simulink model "aerosim_simulink_cosim_demo"  (R2024a)
settings: Solver=FixedStepAuto  StartTime=0.0  StopTime=inf  FixedStep=dt_sec  RelTol=1e-3
values from neighbouring files (symbols this model uses):
  altitude_tgt = 0.0    (= 0)    [load_aerosim_simulink_cosim_demo.m]
  dt_sec = 0.02    [load_aerosim_simulink_cosim_demo.m]
libraries: aerosim_simulink_block_library x6, slpidlib x1
settings Model: Creator=ed  LastModifiedBy=Leo.Wong

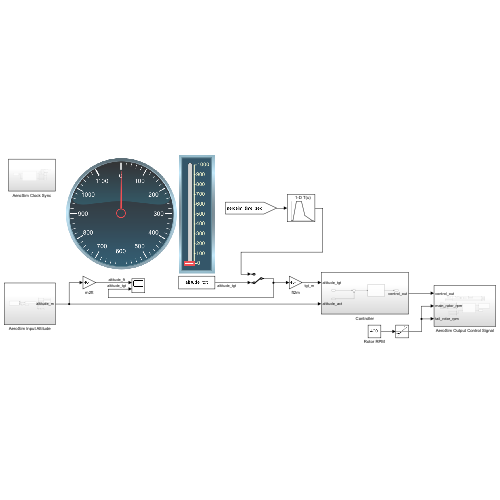
[thumbnail: Simulink's stored preview of the top-level diagram]
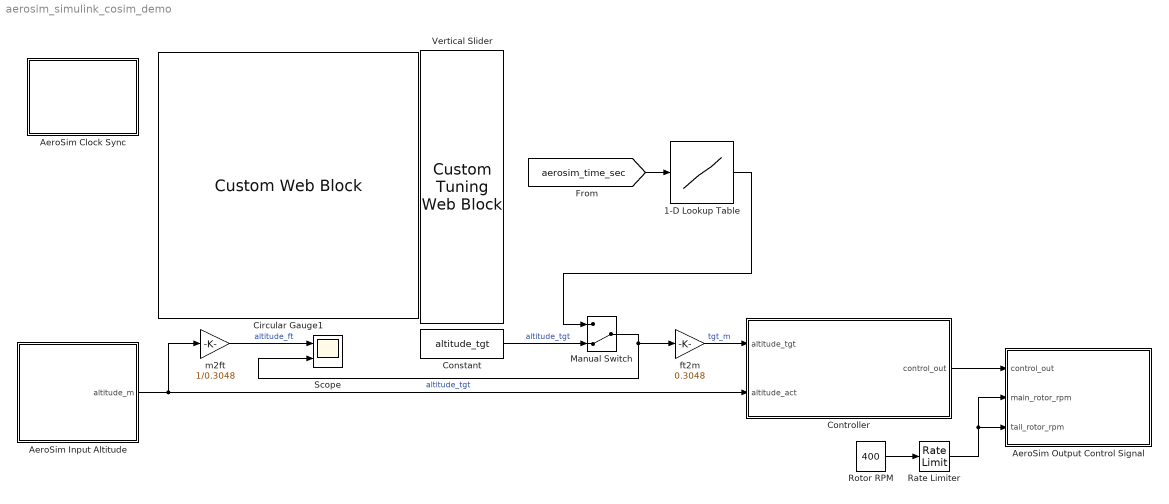
== system aerosim_simulink_cosim_demo ==
  1-D Lookup Table : Lookup_n-D  NumberOfTableDimensions=1  BreakpointsForDimension1=[0;5;15;30;40;60;65]  Table=[0;0;800;800;200;0;0]  ExtrapMethod=Clip  UseLastTableValue=on  InternalRulePriority=Speed  RndMeth=Simplest
  AeroSim Clock Sync : Subsystem  Priority=0
  AeroSim Input Altitude : Subsystem
  AeroSim Output Control Signal : Subsystem
  Circular Gauge1 : CustomWebBlock  LabelPosition=Hide  ShowInitialText=on  Configuration="{\"components\":[{\"name\":\"CircularScaleComponent\",\"settings\":{\"bounds\":{\"max\":1100,\"min\":0,\"tickInterval\":100},\"direction\":\"cw\",\"flipLimits\":0,\"innerRadius\":0.86,\"internalTickHeightScaleFactor\":1,\"labelColor\":[255,255,255],\"labelFont\":{\"font\":\"Arial\",\"fontSize\":12},\"labelRadius\":0.74,\"labelTransparency\":1,\"minorTickHeightScaleFactor\":0.2,\"needleImage\":{\"size\":[200,50],\"src\":\"data:image\\/svg+xml;base64,PD94bWwgdmVyc2lvbj0iMS4wIiBlbmNvZGluZz0idXRmLTgiPz4KPCEtLSBHZW5lcmF0b3I6IEFkb2JlIElsbHVzdHJhdG9yIDI0LjEuMiwgU1ZHIEV4cG9ydCBQbHVnLUluIC4gU1ZHIFZlcnNpb246IDYuMDAgQnVpbGQgMCkgIC0tPgo8c3ZnIHZlcnNpb249IjEuMSIgaWQ9IkxheWVyXzEiIHhtbG5zPSJodHRwOi8vd3d3LnczLm9yZy8yMDAwL3N2ZyIgeG1sbnM6eGxpbms9Imh0dHA6Ly93d3cudzMub3JnLzE5OTkveGxpbmsiIHg9IjBweCIgeT0iMHB4IgoJIHZpZXdCb3g9IjAgMCAyMDAgNTAiIHN0eWxlPSJlbmFibGUtYmFja2dyb3VuZDpuZXcgMCAwIDIwMCA1MDsiIHhtbDpzcGFjZT0icHJlc2VydmUiPgo8c3R5bGUgdHlwZT0idGV4dC9jc3MiPgoJLnN0MHtmaWxsOiNFQzIxMjc7fQo8L3N0eWxlPgo8cGF0aCBjbGFzcz0ic3QwIiBkPSJNMTYyLjgsMTMuN0MxNjksNC40LDE4MS43LDEuOSwxOTEsOC4xczExLjgsMTguOSw1LjYsMjguMnMtMTguOSwxMS44LTI4LjIsNS42bDAsMAoJQzE1OS4xLDM1LjYsMTU2LjYsMjMsMTYyLjgsMTMuN0wxNjIuOCwxMy43eiBNMTY1LjgsMTUuOGMtNS4xLDcuNi0zLjEsMTcuOSw0LjYsMjNjNy42LDUuMSwxNy45LDMuMSwyMy00LjYKCWM1LjEtNy42LDMuMS0xNy45LTQuNi0yM2wwLDBDMTgxLjIsNi4yLDE3MC45LDguMiwxNjUuOCwxNS44eiIvPgo8cGF0aCBjbGFzcz0ic3QwIiBkPSJNMC40LDI1Ljl2LTMuM2wxNTktMi41Yy0wLjcsMi42LTAuNyw1LjIsMCw3LjhMMC40LDI1Ljl6Ii8+CjxjaXJjbGUgY2xhc3M9InN0MCIgY3g9IjE3OS42IiBjeT0iMjQiIHI9IjAuNyIvPgo8L3N2Zz4K\"},\"needleOffset\":[0.18464878250906522,0],\"needleOrientation\":-45,\"needleRotation\":180,\"needleSize\":{\"height\":0.11741692305346914,\"width\":0.46108337545091255},\"outerRadius\":1,\"position\":[0.05,0.05,0.9,0.9],\"referencePoint\":\"auto\",\"scaleAngle\":330,\"scaleAngleOffset\":270,\"scaleColors\":[],\"scaleColorsSize\":0.2,\"scaleDirection\":\"CW\",\"scalePosition\":[0,0,1,1],\"showLabels\":1,\"showMinorTicks\":1,\"showSpanLine\":false,\"showTicks\":true,\"tickColor\":[255,255,255],\"tickTransparency\":1,\"valueBarColor\":[255,255,255],\"valueBarPosition\":[0,0,1,1],\"valueBarSize\":0.2,\"valueBarTransparency\":0.2}},{\"name\":\"BackgroundImageComponent\",\"settings\":{\"image\":{\"size\":[500,500],\"src\":\"data:image\\/svg+xml;base64,PD94bWwgdmVyc2lvbj0iMS4wIiBlbmNvZGluZz0iVVRGLTgiIHN0YW5kYWxvbmU9Im5vIj8+CjxzdmcKICAgeG1sbnM6ZGM9Imh0dHA6Ly9wdXJsLm9yZy9kYy9lbGVtZW50cy8xLjEvIgogICB4bWxuczpjYz0iaHR0cDovL2NyZWF0aXZlY29tbW9ucy5vcmcvbnMjIgogICB4bWxuczpyZGY9Imh0dHA6Ly93d3cudzMub3JnLzE5OTkvMDIvMjItcmRmLXN5bnRheC1ucyMiCiAgIHhtbG5zOnN2Zz0iaHR0cDovL3d3dy53My5vcmcvMjAwMC9zdmciCiAgIHhtbG5zPSJodHRwOi8vd3d3LnczLm9yZy8yMDAwL3N2ZyIKICAgeG1sbnM6 ...(+9964 chars)\"},\"position\":[0,0,1,1],\"scaleMode\":\"0\"}},{\"name\":\"ForegroundImageComponent\",\"settings\":{\"image\":{\"size\":[0,0],\"src\":\"default\",\"srcOrientation\":[]},\"isForeground\":1,\"position\":[0,0,1,1],\"scaleMode\":\"0\"}}],\"settings\":{\"BindingType\":\"signal\",\"aspectRatio\":1.032258064516129,\"backgroundColor\":[0,0,0,\"1\"],\"backgroundOffset\":1,\"backgroundOpacity\":1,\"direction\":\"cw\",\"fixedAspectRatio\":\"on\",\"flipLimits\":0,\"orientation\":\"horizontal\",\"showBackgroundColor\":false,\"value\":0,\"version\":\"R2023a\"},\"type\":\"CircularGauge\"}"
  Constant : Constant  Value=altitude_tgt
  Controller : Subsystem
  Manual Switch : ManualSwitch  CurrentSetting=0
  Rate Limiter : RateLimiter  RisingSlewLimit=50  FallingSlewLimit=-50  SampleTimeMode=inherited
  Rotor RPM : Constant  Value=400
  Scope : Scope  NumInputPorts=2
  Vertical Slider : CustomTuningWebBlock  LabelPosition=Hide  ShowInitialText=on  Configuration="{\"components\":[{\"name\":\"LinearScaleComponent\",\"settings\":{\"bounds\":{\"max\":1000,\"min\":0,\"tickInterval\":100},\"internalTickHeightScaleFactor\":0.5,\"labelColor\":[255,255,200],\"labelFont\":{\"font\":\"Arial\",\"fontSize\":12},\"labelOffset\":0.05,\"labelTransparency\":1,\"needleImage\":{\"size\":[596,842],\"src\":\"data:image\\/svg+xml;base64,PD94bWwgdmVyc2lvbj0iMS4wIiBlbmNvZGluZz0idXRmLTgiPz4NCjwhLS0gR2VuZXJhdG9yOiBBZG9iZSBJbGx1c3RyYXRvciAyNS4wLjAsIFNWRyBFeHBvcnQgUGx1Zy1JbiAuIFNWRyBWZXJzaW9uOiA2LjAwIEJ1aWxkIDApICAtLT4NCjxzdmcgdmVyc2lvbj0iMS4xIg0KCSBpZD0ic3ZnOCIgeG1sbnM6Y2M9Imh0dHA6Ly9jcmVhdGl2ZWNvbW1vbnMub3JnL25zIyIgeG1sbnM6ZGM9Imh0dHA6Ly9wdXJsLm9yZy9kYy9lbGVtZW50cy8xLjEvIiB4bWxuczppbmtzY2FwZT0iaHR0cDovL3d3dy5pbmtzY2FwZS5vcmcvbmFtZXNw ...(+2420 chars)\",\"srcOrientation\":\"horizontal\"},\"needleOffset\":[0.0642123287671233,-0.8044596912521441],\"needleSize\":{\"height\":0.07668067226890757,\"width\":0.4337797619047619},\"position\":[0.03623949579831933,0.2829861111111111,0.6088789682539683,0.9196428571428571],\"referencePoint\":\"auto\",\"scaleColors\":[],\"scaleColorsSize\":0.2,\"scaleDirection\":\"BT\",\"showLabels\":1,\"showMinorTicks\":0,\"showSpanLine\":1,\"showTicks\":1,\"tickColor\":[252,252,197],\"tickTransparency\":1,\"valueBarColor\":[0,114,189],\"valueBarOffset\":-0.27,\"valueBarSize\":0.1,\"valueBarTransparency\":1}},{\"name\":\"BackgroundImageComponent\",\"settings\":{\"image\":{\"size\":[380,101],\"src\":\"data:image\\/svg+xml;base64,PHN2ZyB4bWxucz0iaHR0cDovL3d3dy53My5vcmcvMjAwMC9zdmciIHhtbG5zOnhsaW5rPSJodHRwOi8vd3d3LnczLm9yZy8xOTk5L3hsaW5rIiB2aWV3Qm94PSIwIDAgMzgwIDEwMSI+PGRlZnM+PHN0eWxlPi5jbHMtMXtmaWxsOiMwMDJiNDI7fS5jbHMtMntmaWxsOiM0MjcwODI7fS5jbHMtM3tmaWxsOnVybCgjcmFkaWFsLWdyYWRpZW50KTt9LmNscy00e2ZpbGw6I2M4YzhjODtzdHJva2U6IzAwMDt9PC9zdHlsZT48cmFkaWFsR3JhZGllbnQgaWQ9InJhZGlhbC1ncmFkaWVudCIgY3g9IjE5MCIgY3k9IjUwLjUiIHI9IjI2OS4yMSIgZ3JhZGllbnRVbml0cz0idXNlclNwYWNlT25Vc2UiPjxzdG9wIG9mZnNldD0iMC4wMSIgc3RvcC1jb2xvcj0iIzNlNGY1OCIvPjxzdG9wIG9mZnNldD0iMC4wNiIgc3RvcC1jb2xvcj0iIzQ0NTc2MSIvPjxzdG9wIG9mZnNldD0iMC4xNSIgc3RvcC1jb2xvcj0iIzU1NmE3NiIvPjxzdG9wIG9mZnNldD0iMC4yNSIgc3RvcC1jb2xvcj0iIzZkODg5NSIvPjxzdG9wIG9mZnNldD0iMC4zOCIgc3RvcC1jb2xvcj0iIzhmYjJjMyIvPjxzdG9wIG9mZnNldD0iMC41MiIgc3RvcC1jb2xvcj0iI2I2ZTRmYSIvPjxzdG9wIG9mZnNldD0iMSIgc3RvcC1jb2xvcj0iIzE1NDY1NyIvPjwvcmFkaWFsR3JhZGllbnQ+PC9kZWZzPjxnIGlkPSJmcmFtZSI+PGcgaWQ9IkxheWVyXzIiIGRhdGEtbmFtZT0iTGF5ZXIgMiI+PGcgaWQ9IkxheWVyXzEtMiIgZGF0YS1uYW1lPSJMYXllciAxLTIiPjxyZWN0IGlkPSJyZWN0MTAzNiIgY2xhc3M9ImNscy0xIiB4PSIxMSIgeT0iMTEiIHdpZHRoPSIzNTgiIGhlaWdodD0iNzkiLz48cGF0aCBpZD0icGF0aDEwMzgiIGNsYXNzPSJjbHMtMiIgZD0iTTgsOFY5M0gzNzJWOFpNMzY5LDkwSDExVjExSDM2OVoiLz48cGF0aCBpZD0icGF0aDEwNDAiIGNsYXNzPSJjbHMtMyIgZD0iTTAsMFYxMDFIMzgwVjBaTTM3Miw5M0g4VjhIMzcyWiIvPjwvZz48L2c+PC9nPjxnIGlkPSJ0cmFjayI+PHBhdGggaWQ9InJlY3QxNjExIiBjbGFzcz0iY2xzLTQiIGQ9Ik0zMy4zNywyNi41OUgzNDYuNjNjNCwwLDcuMjUsMi42LDcuMjUsNS44MWgwYzAsMy4yMS0zLjI1LDUuODItNy4yNSw1LjgySDMzLjM3Yy00LDAtNy4yNS0yLjYxLTcuMjUtNS44MmgwQzI2LjEyLDI5LjE5LDI5LjM3LDI2LjU5LDMzLjM3LDI2LjU5WiIvPjwvZz48L3N2Zz4=\",\"srcOrientation\":\"horizontal\"},\"position\":[0,0,1,1],\"scaleMode\":\"0\"}},{\"name\":\"ForegroundImageComponent\",\"settings\":{\"image\":{\"size\":[0,0],\"src\":\"default\",\"srcOrientation\":[]},\"isForeground\":1,\"position\":[0,0,1,1],\"scaleMode\":\"0\"}}],\"settings\":{\"BindingType\":\"param\",\"aspectRatio\":3.7777777777777777,\"backgroundColor\":[0,0,0,\"1\"],\"backgroundOffset\":0,\"backgroundOpacity\":1,\"fixedAspectRatio\":\"off\",\"foregroundColor\":[252,252,196],\"orientation\":\"vertical\",\"showBackgroundColor\":false,\"value\":0,\"version\":\"R2023a\"},\"type\":\"LinearGauge\"}"
  ft2m : Gain  Gain=0.3048
  m2ft : Gain  Gain=1/0.3048
  wires:
  Manual Switch/1 -> ft2m/1, Scope/2  "altitude_tgt"
  AeroSim Input Altitude/1(altitude_m) -> m2ft/1, Controller/2(altitude_act)
  m2ft/1 -> Scope/1  "altitude_ft"
  ft2m/1 -> Controller/1(altitude_tgt)  "tgt_m"
  Controller/1(control_out) -> AeroSim Output Control Signal/1(control_out)
  [aerosim_time_sec] -> 1-D Lookup Table/1
  Constant/1 -> Manual Switch/2  "altitude_tgt"
  1-D Lookup Table/1 -> Manual Switch/1
  Rotor RPM/1 -> Rate Limiter/1
  Rate Limiter/1 -> AeroSim Output Control Signal/2(main_rotor_rpm), AeroSim Output Control Signal/3(tail_rotor_rpm)

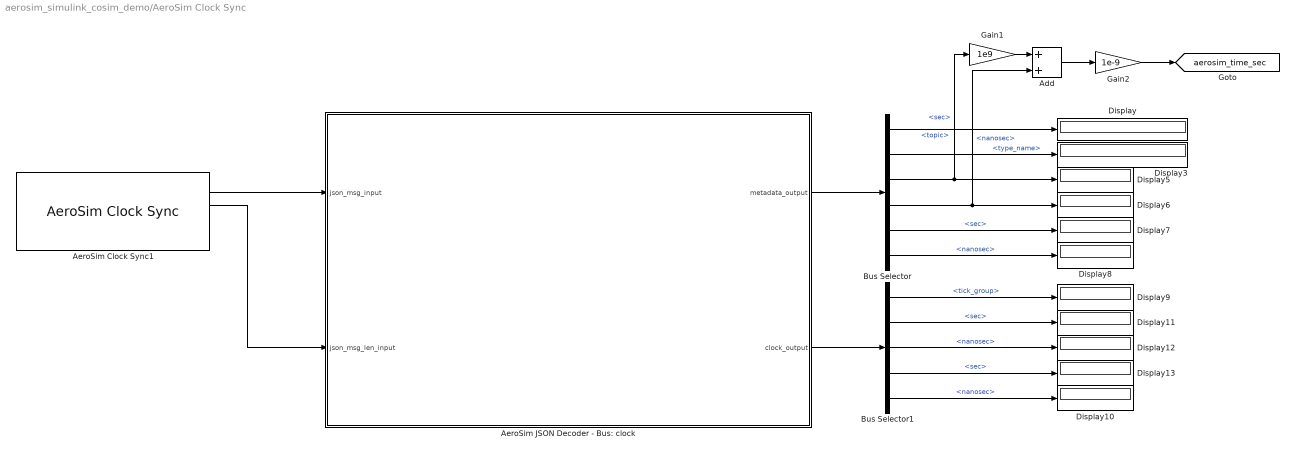
== system aerosim_simulink_cosim_demo/AeroSim Clock Sync ==
  Add : Sum
  AeroSim Clock Sync1 : aerosim_simulink_block_library/AeroSim Clock Sync  sfpBrokers='127.0.0.1:9092'  sfpStartCmdTimeout=30  sfpClockMsgTimeout=10  sfpMsgLen=5000  sfpKeyLen=32  sfpOutputTimestamp=on  sfpTS=0  sfpConf=|  sfpTopicConf=auto.offset.reset=latest
      | client.id=sl_kafka_consumer
      | message.copy.max.bytes=65535
      | broker.address.family=v4
      | socket.nagle.disable=true
  AeroSim JSON Decoder - Bus: clock : Subsystem
  Bus Selector : BusSelector  OutputSignals=topic,type_name,timestamp_sim.sec,timestamp_sim.nanosec,timestamp_platform.sec,timestamp_platform.nanosec
  Bus Selector1 : BusSelector  OutputSignals=tick_group,timestamp_real.sec,timestamp_real.nanosec,timestamp_sim.sec,timestamp_sim.nanosec
  Display{,3,5..13} (11 alike) : Display
  Gain1 : Gain  Gain=1e9
  Gain2 : Gain  Gain=1e-9
  tag scope: aerosim_time_sec=global
  wires:
  AeroSim Clock Sync1/2 -> AeroSim JSON Decoder - Bus: clock/1(json_msg_input)
  AeroSim Clock Sync1/3 -> AeroSim JSON Decoder - Bus: clock/2(json_msg_len_input)
  Bus Selector/6 -> Display8/1  "<nanosec>"
  Bus Selector1/5 -> Display10/1  "<nanosec>"
  Bus Selector1/3 -> Display12/1  "<nanosec>"
  Bus Selector/2 -> Display3/1  "<type_name>"
  Bus Selector1/2 -> Display11/1  "<sec>"
  Bus Selector/3 -> Gain1/1, Display5/1  "<sec>"
  Bus Selector/5 -> Display7/1  "<sec>"
  AeroSim JSON Decoder - Bus: clock/1(metadata_output) -> Bus Selector/1
  Bus Selector1/4 -> Display13/1  "<sec>"
  AeroSim JSON Decoder - Bus: clock/2(clock_output) -> Bus Selector1/1
  Bus Selector1/1 -> Display9/1  "<tick_group>"
  Bus Selector/1 -> Display/1  "<topic>"
  Bus Selector/4 -> Add/2, Display6/1  "<nanosec>"
  Add/1 -> Gain2/1
  Gain2/1 -> [aerosim_time_sec]
  Gain1/1 -> Add/1

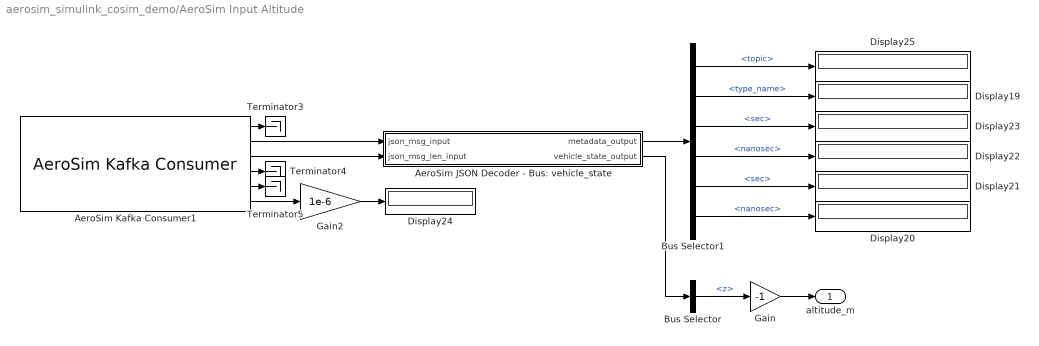
== system aerosim_simulink_cosim_demo/AeroSim Input Altitude ==
  AeroSim JSON Decoder - Bus: vehicle_state : Subsystem
  AeroSim Kafka Consumer1 : aerosim_simulink_block_library/AeroSim Kafka Consumer  sfpBrokers='127.0.0.1:9092'  sfpTopic='aerosim.actor1.vehicle_state'  sfpGroup='aerosim.simulink'  sfpMsgLen=1024  sfpKeyLen=32  sfpOutputTimestamp=on  sfpTS=0  sfpConf=|  sfpTopicConf=compression.level=-1
      | client.id=sl_kafka_consumer
      | message.copy.max.bytes=65535
      | broker.address.family=v4
      | socket.nagle.disable=true
  Bus Selector : BusSelector  OutputSignals=state.pose.position.z
  Bus Selector1 : BusSelector  OutputSignals=topic,type_name,timestamp_sim.sec,timestamp_sim.nanosec,timestamp_platform.sec,timestamp_platform.nanosec
  Display{19..25} (7 alike) : Display
  Gain : Gain  Gain=-1
  Gain2 : Gain  Gain=1e-6
  Terminator3 : Terminator
  Terminator4 : Terminator
  Terminator5 : Terminator
  altitude_m : Outport
  wires:
  AeroSim Kafka Consumer1/1 -> Terminator3/1
  Gain2/1 -> Display24/1
  AeroSim Kafka Consumer1/6 -> Gain2/1
  AeroSim Kafka Consumer1/4 -> Terminator4/1
  AeroSim Kafka Consumer1/5 -> Terminator5/1
  AeroSim Kafka Consumer1/2 -> AeroSim JSON Decoder - Bus: vehicle_state/1(json_msg_input)
  AeroSim Kafka Consumer1/3 -> AeroSim JSON Decoder - Bus: vehicle_state/2(json_msg_len_input)
  Bus Selector1/3 -> Display23/1  "<sec>"
  AeroSim JSON Decoder - Bus: vehicle_state/1(metadata_output) -> Bus Selector1/1
  Bus Selector1/6 -> Display20/1  "<nanosec>"
  Bus Selector1/1 -> Display25/1  "<topic>"
  Bus Selector1/4 -> Display22/1  "<nanosec>"
  Bus Selector1/5 -> Display21/1  "<sec>"
  Bus Selector1/2 -> Display19/1  "<type_name>"
  AeroSim JSON Decoder - Bus: vehicle_state/2(vehicle_state_output) -> Bus Selector/1
  Bus Selector/1 -> Gain/1  "<z>"
  Gain/1 -> altitude_m/1

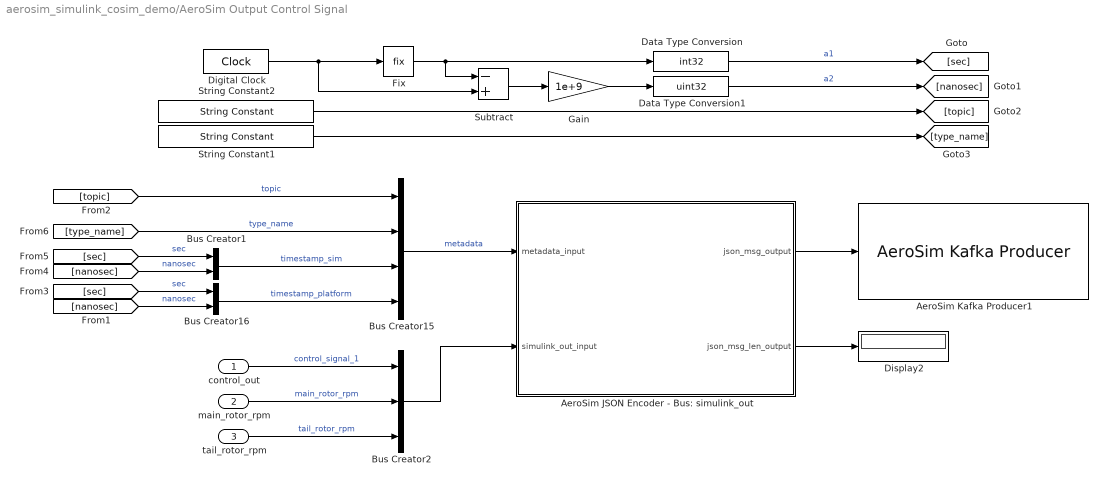
== system aerosim_simulink_cosim_demo/AeroSim Output Control Signal ==
  control_out : Inport
  main_rotor_rpm : Inport  Port=2
  tail_rotor_rpm : Inport  Port=3
  AeroSim JSON Encoder - Bus: simulink_out : Subsystem
  AeroSim Kafka Producer1 : aerosim_simulink_block_library/AeroSim Kafka Producer  sfpBrokers='127.0.0.1:9092'  sfpTopic='aerosim.simulink_out'  sfpKeyAsInput=off  sfpKeyAsInputLen=16  sfpKey='mykey'  sfpMsgLen=1024  sfpTS=0  sfpExtTimestamp=off  sfpConf=|  sfpTopicConf=compression.level=-1
      | client.id=sl_kafka_producer
      | message.copy.max.bytes=65535
      | broker.address.family=v4
      | socket.nagle.disable=true
      | linger.ms=0
      | enable.idempotence=true
      | acks=all
  Bus Creator1 : BusCreator  Inputs=2  OutDataTypeStr=Bus: timestamp_sim
  Bus Creator15 : BusCreator  Inputs=4  OutDataTypeStr=Bus: metadata
  Bus Creator16 : BusCreator  Inputs=2  OutDataTypeStr=Bus: timestamp_platform
  Bus Creator2 : BusCreator  Inputs=3  OutDataTypeStr=Bus: simulink_out
  Data Type Conversion : DataTypeConversion  OutDataTypeStr=int32  SaturateOnIntegerOverflow=off  RndMeth=Floor
  Data Type Conversion1 : DataTypeConversion  OutDataTypeStr=uint32  SaturateOnIntegerOverflow=off  RndMeth=Floor
  Digital Clock : DigitalClock  SampleTime=dt_sec
  Display2 : Display
  Fix : Rounding  Operator=fix
  Gain : Gain  Gain=1e+9
  String Constant1 : StringConstant  String="\"aerosim::types::JsonData\""
  String Constant2 : StringConstant  String="\"aerosim.simulink_out\""
  Subtract : Sum  Inputs=-+
  wires:
  [nanosec] -> Bus Creator1/2  "nanosec"
  Bus Creator1/1 -> Bus Creator15/3  "timestamp_sim"
  [type_name] -> Bus Creator15/2  "type_name"
  Fix/1 -> Data Type Conversion/1, Subtract/1
  [topic] -> Bus Creator15/1  "topic"
  String Constant1/1 -> [type_name]
  Data Type Conversion1/1 -> [nanosec]  "a2"
  Digital Clock/1 -> Subtract/2, Fix/1
  [sec] -> Bus Creator1/1  "sec"
  Data Type Conversion/1 -> [sec]  "a1"
  String Constant2/1 -> [topic]
  Gain/1 -> Data Type Conversion1/1
  Bus Creator16/1 -> Bus Creator15/4  "timestamp_platform"
  [sec] -> Bus Creator16/1  "sec"
  Bus Creator15/1 -> AeroSim JSON Encoder - Bus: simulink_out/1(metadata_input)  "metadata"
  [nanosec] -> Bus Creator16/2  "nanosec"
  Subtract/1 -> Gain/1
  AeroSim JSON Encoder - Bus: simulink_out/1(json_msg_output) -> AeroSim Kafka Producer1/1
  AeroSim JSON Encoder - Bus: simulink_out/2(json_msg_len_output) -> Display2/1
  Bus Creator2/1 -> AeroSim JSON Encoder - Bus: simulink_out/2(simulink_out_input)
  control_out/1 -> Bus Creator2/1  "control_signal_1"
  main_rotor_rpm/1 -> Bus Creator2/2  "main_rotor_rpm"
  tail_rotor_rpm/1 -> Bus Creator2/3  "tail_rotor_rpm"

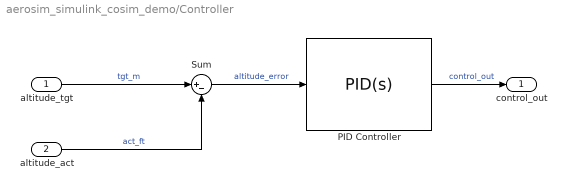
== system aerosim_simulink_cosim_demo/Controller ==
  altitude_tgt : Inport
  altitude_act : Inport  Port=2
  PID Controller : slpidlib/PID Controller  Controller=PID  Form=Parallel  TimeDomain=Continuous-time  UseExternalTs=off  SampleTime=-1  IntegratorMethod=Forward Euler  FilterMethod=Forward Euler  ControllerParametersSource=internal  P=40  I=0  UseKiTs=off  D=40  UseExternalDerivativeSource=off  N=100  UseFilter=on  TunerSelectOption=Transfer Function Based (PID Tuner App)  InitialConditionSource=internal  InitialConditionForIntegrator=0  InitialConditionForFilter=0  DifferentiatorICPrevScaledInput=0  ExternalReset=none  TrackingMode=off  Kt=1  LimitOutput=on  SatLimitsSource=internal  UpperSaturationLimit=20  LowerSaturationLimit=0  LinearizeAsGain=on  AntiWindupMode=clamping  Kb=1  LimitIntegrator=off  UpperIntegratorSaturationLimit=inf  LowerIntegratorSaturationLimit=-inf  POutMin=[]  POutMax=[]  IOutMin=[]  IOutMax=[]  DOutMin=[]  DOutMax=[]  NOutMin=[]  NOutMax=[]  SumOutMin=[]  SumOutMax=[]  SaturationOutMin=[]  SaturationOutMax=[]  PParamMin=[]  PParamMax=[]  IParamMin=[]  IParamMax=[]  DParamMin=[]  DParamMax=[]  NParamMin=[]  NParamMax=[]  KbParamMin=[]  KbParamMax=[]  KtParamMin=[]  KtParamMax=[]  KbOutMin=[]  KbOutMax=[]  KtOutMin=[]  KtOutMax=[]  IntegratorOutMin=[]  IntegratorOutMax=[]  FilterOutMin=[]  FilterOutMax=[]  SumI1OutMin=[]  SumI1OutMax=[]  SumI2OutMin=[]  SumI2OutMax=[]  SumI3OutMin=[]  SumI3OutMax=[]  SumI4OutMin=[]  SumI4OutMax=[]  SumDOutMin=[]  SumDOutMax=[]  DifferentiatorOutMin=[]  DifferentiatorOutMax=[]  FilterDiffOutCoefMin=[]  FilterDiffOutCoefMax=[]  ReciprocalOutMin=[]  ReciprocalOutMax=[]  SumDenOutMin=[]  SumDenOutMax=[]  SumNumOutMin=[]  SumNumOutMax=[]  DivideOutMin=[]  DivideOutMax=[]  UdiffTsProdOutMin=[]  UdiffTsProdOutMax=[]  NTsProdOutMin=[]  NTsProdOutMax=[]  UintegralTsProdOutMin=[]  UintegralTsProdOutMax=[]  UngainTsProdOutMin=[]  UngainTsProdOutMax=[]  ClampingZeroOutDataTypeStr=Inherit: Inherit via back propagation  ClampingZeroOutMin=[]  ClampingZeroOutMax=[]  FilterDenConstantOutDataTypeStr=Inherit: Inherit via back propagation  FilterDenConstantOutMin=[]  FilterDenConstantOutMax=[]  PCopyOutDataTypeStr=Inherit: Inherit via back propagation  PCopyOutMin=[]  PCopyOutMax=[]  NCopyOutDataTypeStr=Inherit: Inherit via back propagation  NCopyOutMin=[]  NCopyOutMax=[]  IntegratorContinuousStateAttributes=''  IntegratorStateMustResolveToSignalObject=off  IntegratorRTWStateStorageClass=Auto  FilterContinuousStateAttributes=''  FilterStateMustResolveToSignalObject=off  FilterRTWStateStorageClass=Auto  ParallelPVariant=InternalParameters  IdealPVariant=Disabled  IVariant=InternalParameters  DVariant=InternalParameters  IntegratorVariant=Continuous  SatVariant=Enabled  AWVariant=ContClampingParallel  PCopyVariant=Disabled  TRVariant=Disabled  FdbkBlocksVariant=Forward  IdealPFdbkVariant=Disabled  SatFdbkVariant=Disabled  DerivativeFilterVariant=ContFilter  NVariant=InternalParameters  NCopyVariant=Disabled  FilterICVariant=InternalICsFilter  IntegratorICVariant=InternalICs  ExternalResetVariant=Disabled  TRSumVariant=Passthrough  SumFdbkVariant=Disabled  SumVariant=Sum_PID  TsampFilterVariant=InternalTs  TsampNgainVariant=Passthrough  TsampIntegralVariant=Disabled_SignalSpec  ExternalSaturationOutDataTypeStr=Inherit: Same as second input  DerivativeSourceVariant=ErrorSignal
  Sum : Sum  Inputs=|+-
  control_out : Outport
  wires:
  PID Controller/1 -> control_out/1  "control_out"
  Sum/1 -> PID Controller/1  "altitude_error"
  altitude_act/1 -> Sum/2  "act_ft"
  altitude_tgt/1 -> Sum/1  "tgt_m"

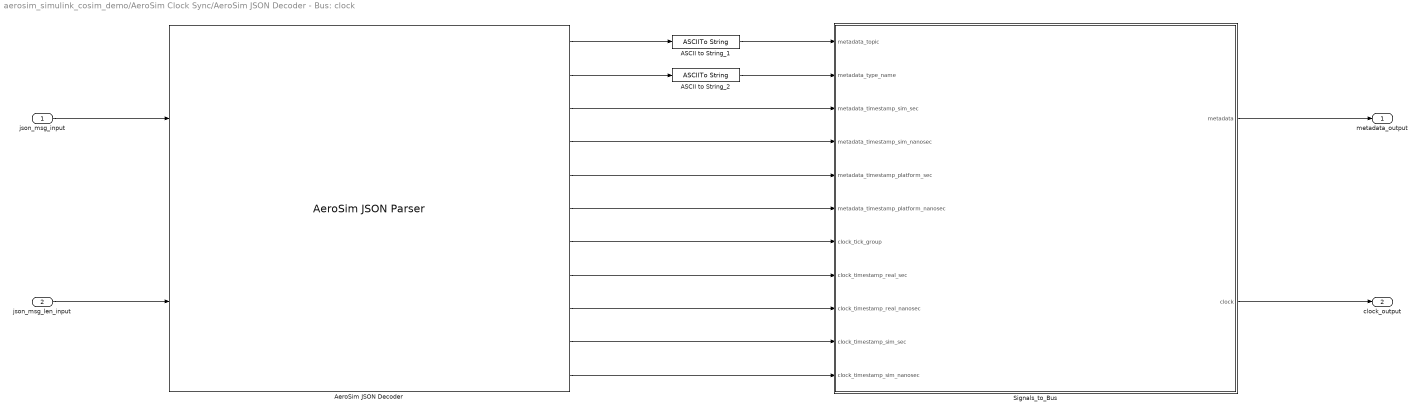
== system aerosim_simulink_cosim_demo/AeroSim Clock Sync/AeroSim JSON Decoder - Bus: clock ==
  json_msg_input : Inport
  json_msg_len_input : Inport  Port=2
  ASCII to String_1 : ASCIIToString
  ASCII to String_2 : ASCIIToString
  AeroSim JSON Decoder : aerosim_simulink_block_library/AeroSim JSON Parser  sfpDirection=Decode  sfpLength=5000  sfpFields={'metadata.topic','metadata.type_name','metadata.timestamp_sim.sec','metadata.timestamp_sim.nanosec','metadata.timestamp_platform.sec','metadata.timestamp_platform.nanosec','clock.tick_group','clock.timestamp_real.sec','clock.timestamp_real.nanosec','clock.timestamp_sim.sec','clock.timestamp_sim.nanosec'}  sfpFieldTypes={'string','string','int32','uint32','int32','uint32','int32','int32','uint32','int32','uint32'}  sfpOutLength=on  sfpInLength=on
  Signals_to_Bus : MATLAB Function  TreatAsAtomicUnit=on  SystemSampleTime=dt_sec
  metadata_output : Outport  OutDataTypeStr=Bus: metadata
  clock_output : Outport  Port=2  OutDataTypeStr=Bus: clock
  wires:
  AeroSim JSON Decoder/1 -> ASCII to String_1/1
  ASCII to String_1/1 -> Signals_to_Bus/1(metadata_topic)
  AeroSim JSON Decoder/2 -> ASCII to String_2/1
  ASCII to String_2/1 -> Signals_to_Bus/2(metadata_type_name)
  AeroSim JSON Decoder/3 -> Signals_to_Bus/3(metadata_timestamp_sim_sec)
  AeroSim JSON Decoder/4 -> Signals_to_Bus/4(metadata_timestamp_sim_nanosec)
  AeroSim JSON Decoder/5 -> Signals_to_Bus/5(metadata_timestamp_platform_sec)
  AeroSim JSON Decoder/6 -> Signals_to_Bus/6(metadata_timestamp_platform_nanosec)
  AeroSim JSON Decoder/7 -> Signals_to_Bus/7(clock_tick_group)
  AeroSim JSON Decoder/8 -> Signals_to_Bus/8(clock_timestamp_real_sec)
  AeroSim JSON Decoder/9 -> Signals_to_Bus/9(clock_timestamp_real_nanosec)
  AeroSim JSON Decoder/10 -> Signals_to_Bus/10(clock_timestamp_sim_sec)
  AeroSim JSON Decoder/11 -> Signals_to_Bus/11(clock_timestamp_sim_nanosec)
  json_msg_input/1 -> AeroSim JSON Decoder/1
  json_msg_len_input/1 -> AeroSim JSON Decoder/2
  Signals_to_Bus/1(metadata) -> metadata_output/1
  Signals_to_Bus/2(clock) -> clock_output/1

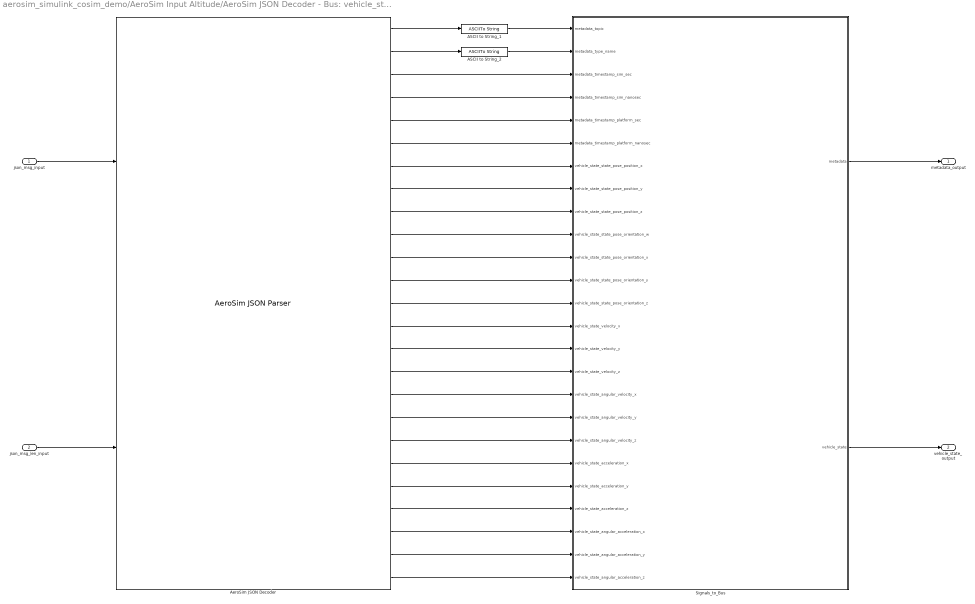
== system aerosim_simulink_cosim_demo/AeroSim Input Altitude/AeroSim JSON Decoder - Bus: vehicle_state ==
  json_msg_input : Inport
  json_msg_len_input : Inport  Port=2
  ASCII to String_1 : ASCIIToString
  ASCII to String_2 : ASCIIToString
  AeroSim JSON Decoder : aerosim_simulink_block_library/AeroSim JSON Parser  sfpDirection=Decode  sfpLength=1024  sfpFields={'metadata.topic','metadata.type_name','metadata.timestamp_sim.sec','metadata.timestamp_sim.nanosec','metadata.timestamp_platform.sec','metadata.timestamp_platform.nanosec','vehicle_state.state.pose.position.x','vehicle_state.state.pose.position.y','vehicle_state.state.pose.position.z','vehicle_state.state.pose.orientation.w','vehicle_state.state.pose.orientation.x','vehicle_state.state.pose.orientation.y','vehicle_state.state.pose.orientation.z','vehicle_state.velocity.x','vehicle_state.velocity.y','vehicle_state.velocity.z','vehicle_state.angular_velocity.x','vehicle_state.angular_velocity.y','vehicle_state.angular_velocity.z','vehicle_state.acceleration.x','vehicle_state.acceleration.y','vehicle_state.acceleration.z','vehicle_state.angular_acceleration.x','vehicle_state.angular_acceleration.y','vehicle_state.angular_acceleration.z'}  sfpFieldTypes={'string','string','int32','uint32','int32','uint32','double','double','double','double','double','double','double','double','double','double','double','double','double','double','double','double','double','double','double'}  sfpOutLength=on  sfpInLength=on
  Signals_to_Bus : MATLAB Function  TreatAsAtomicUnit=on  SystemSampleTime=dt_sec
  metadata_output : Outport  OutDataTypeStr=Bus: metadata
  vehicle_state_output : Outport  Port=2  OutDataTypeStr=Bus: vehicle_state
  wires:
  AeroSim JSON Decoder/1 -> ASCII to String_1/1
  ASCII to String_1/1 -> Signals_to_Bus/1(metadata_topic)
  AeroSim JSON Decoder/2 -> ASCII to String_2/1
  ASCII to String_2/1 -> Signals_to_Bus/2(metadata_type_name)
  AeroSim JSON Decoder/3 -> Signals_to_Bus/3(metadata_timestamp_sim_sec)
  AeroSim JSON Decoder/4 -> Signals_to_Bus/4(metadata_timestamp_sim_nanosec)
  AeroSim JSON Decoder/5 -> Signals_to_Bus/5(metadata_timestamp_platform_sec)
  AeroSim JSON Decoder/6 -> Signals_to_Bus/6(metadata_timestamp_platform_nanosec)
  AeroSim JSON Decoder/7 -> Signals_to_Bus/7(vehicle_state_state_pose_position_x)
  AeroSim JSON Decoder/8 -> Signals_to_Bus/8(vehicle_state_state_pose_position_y)
  AeroSim JSON Decoder/9 -> Signals_to_Bus/9(vehicle_state_state_pose_position_z)
  AeroSim JSON Decoder/10 -> Signals_to_Bus/10(vehicle_state_state_pose_orientation_w)
  AeroSim JSON Decoder/11 -> Signals_to_Bus/11(vehicle_state_state_pose_orientation_x)
  AeroSim JSON Decoder/12 -> Signals_to_Bus/12(vehicle_state_state_pose_orientation_y)
  AeroSim JSON Decoder/13 -> Signals_to_Bus/13(vehicle_state_state_pose_orientation_z)
  AeroSim JSON Decoder/14 -> Signals_to_Bus/14(vehicle_state_velocity_x)
  AeroSim JSON Decoder/15 -> Signals_to_Bus/15(vehicle_state_velocity_y)
  AeroSim JSON Decoder/16 -> Signals_to_Bus/16(vehicle_state_velocity_z)
  AeroSim JSON Decoder/17 -> Signals_to_Bus/17(vehicle_state_angular_velocity_x)
  AeroSim JSON Decoder/18 -> Signals_to_Bus/18(vehicle_state_angular_velocity_y)
  AeroSim JSON Decoder/19 -> Signals_to_Bus/19(vehicle_state_angular_velocity_z)
  AeroSim JSON Decoder/20 -> Signals_to_Bus/20(vehicle_state_acceleration_x)
  AeroSim JSON Decoder/21 -> Signals_to_Bus/21(vehicle_state_acceleration_y)
  AeroSim JSON Decoder/22 -> Signals_to_Bus/22(vehicle_state_acceleration_z)
  AeroSim JSON Decoder/23 -> Signals_to_Bus/23(vehicle_state_angular_acceleration_x)
  AeroSim JSON Decoder/24 -> Signals_to_Bus/24(vehicle_state_angular_acceleration_y)
  AeroSim JSON Decoder/25 -> Signals_to_Bus/25(vehicle_state_angular_acceleration_z)
  json_msg_input/1 -> AeroSim JSON Decoder/1
  json_msg_len_input/1 -> AeroSim JSON Decoder/2
  Signals_to_Bus/1(metadata) -> metadata_output/1
  Signals_to_Bus/2(vehicle_state) -> vehicle_state_output/1

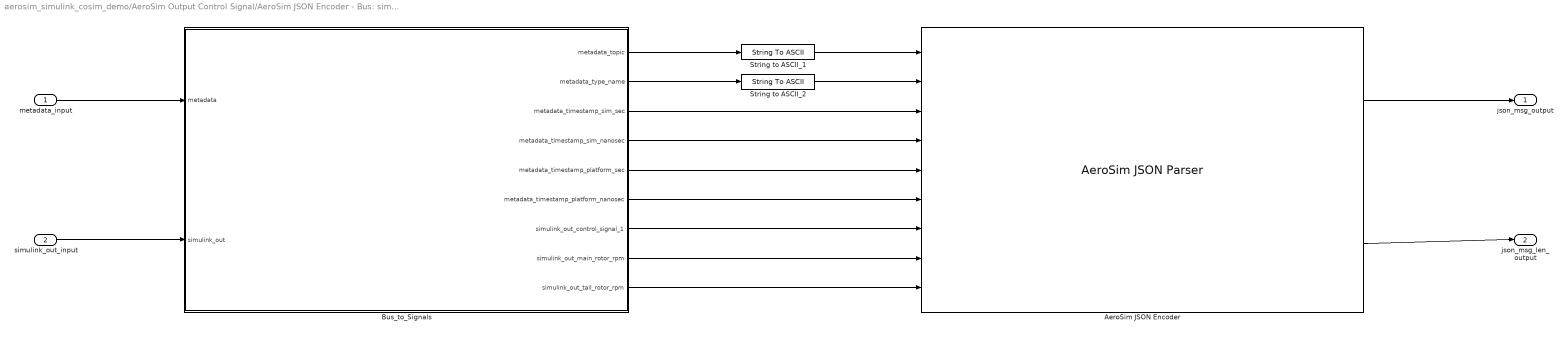
== system aerosim_simulink_cosim_demo/AeroSim Output Control Signal/AeroSim JSON Encoder - Bus: simulink_out ==
  metadata_input : Inport  OutDataTypeStr=Bus: metadata
  simulink_out_input : Inport  Port=2  OutDataTypeStr=Bus: simulink_out
  AeroSim JSON Encoder : aerosim_simulink_block_library/AeroSim JSON Parser  sfpDirection=Encode  sfpLength=1024  sfpFields={'metadata.topic','metadata.type_name','metadata.timestamp_sim.sec','metadata.timestamp_sim.nanosec','metadata.timestamp_platform.sec','metadata.timestamp_platform.nanosec','simulink_out.control_signal_1','simulink_out.main_rotor_rpm','simulink_out.tail_rotor_rpm'}  sfpFieldTypes={'string','string','int32','uint32','int32','uint32','double','double','double'}  sfpOutLength=on  sfpInLength=on
  Bus_to_Signals : MATLAB Function  TreatAsAtomicUnit=on  SystemSampleTime=dt_sec
  String to ASCII_1 : StringToASCII  OutputVectorSize=1024
  String to ASCII_2 : StringToASCII  OutputVectorSize=1024
  json_msg_output : Outport
  json_msg_len_output : Outport  Port=2
  wires:
  Bus_to_Signals/1(metadata_topic) -> String to ASCII_1/1
  String to ASCII_1/1 -> AeroSim JSON Encoder/1
  Bus_to_Signals/2(metadata_type_name) -> String to ASCII_2/1
  String to ASCII_2/1 -> AeroSim JSON Encoder/2
  Bus_to_Signals/3(metadata_timestamp_sim_sec) -> AeroSim JSON Encoder/3
  Bus_to_Signals/4(metadata_timestamp_sim_nanosec) -> AeroSim JSON Encoder/4
  Bus_to_Signals/5(metadata_timestamp_platform_sec) -> AeroSim JSON Encoder/5
  Bus_to_Signals/6(metadata_timestamp_platform_nanosec) -> AeroSim JSON Encoder/6
  Bus_to_Signals/7(simulink_out_control_signal_1) -> AeroSim JSON Encoder/7
  AeroSim JSON Encoder/1 -> json_msg_output/1
  AeroSim JSON Encoder/2 -> json_msg_len_output/1
  metadata_input/1 -> Bus_to_Signals/1(metadata)
  simulink_out_input/1 -> Bus_to_Signals/2(simulink_out)
  Bus_to_Signals/8(simulink_out_main_rotor_rpm) -> AeroSim JSON Encoder/8
  Bus_to_Signals/9(simulink_out_tail_rotor_rpm) -> AeroSim JSON Encoder/9

== matlab function aerosim_simulink_cosim_demo/AeroSim Clock Sync/AeroSim JSON Decoder - Bus: clock/Signals_to_Bus ==
  data: metadata_topic input string; metadata output Bus: metadata; metadata_type_name input string; metadata_timestamp_sim_sec input int32; metadata_timestamp_sim_nanosec input uint32; metadata_timestamp_platform_sec input int32; metadata_timestamp_platform_nanosec input uint32; clock_tick_group input int32; clock_timestamp_real_sec input int32; clock_timestamp_real_nanosec input uint32; clock_timestamp_sim_sec input int32; clock_timestamp_sim_nanosec input uint32; clock output Bus: clock
function [metadata, clock] = signals_to_bus(...
	metadata_topic, ...
	metadata_type_name, ...
	metadata_timestamp_sim_sec, ...
	metadata_timestamp_sim_nanosec, ...
	metadata_timestamp_platform_sec, ...
	metadata_timestamp_platform_nanosec, ...
	clock_tick_group, ...
	clock_timestamp_real_sec, ...
	clock_timestamp_real_nanosec, ...
	clock_timestamp_sim_sec, ...
	clock_timestamp_sim_nanosec )

metadata.topic = metadata_topic;
metadata.type_name = metadata_type_name;
metadata.timestamp_sim.sec = metadata_timestamp_sim_sec;
metadata.timestamp_sim.nanosec = metadata_timestamp_sim_nanosec;
metadata.timestamp_platform.sec = metadata_timestamp_platform_sec;
metadata.timestamp_platform.nanosec = metadata_timestamp_platform_nanosec;
clock.tick_group = clock_tick_group;
clock.timestamp_real.sec = clock_timestamp_real_sec;
clock.timestamp_real.nanosec = clock_timestamp_real_nanosec;
clock.timestamp_sim.sec = clock_timestamp_sim_sec;
clock.timestamp_sim.nanosec = clock_timestamp_sim_nanosec;

== matlab function aerosim_simulink_cosim_demo/AeroSim Input Altitude/AeroSim JSON Decoder - Bus: vehicle_state/Signals_to_Bus ==
  data: metadata_topic input string; metadata output Bus: metadata; metadata_type_name input string; metadata_timestamp_sim_sec input int32; metadata_timestamp_sim_nanosec input uint32; metadata_timestamp_platform_sec input int32; metadata_timestamp_platform_nanosec input uint32; vehicle_state_state_pose_position_x input double; vehicle_state_state_pose_position_y input double; vehicle_state_state_pose_position_z input double; vehicle_state_state_pose_orientation_w input double; vehicle_state_state_pose_orientation_x input double; vehicle_state_state_pose_orientation_y input double; vehicle_state_state_pose_orientation_z input double; vehicle_state_velocity_x input double; vehicle_state_velocity_y input double; vehicle_state_velocity_z input double; vehicle_state_angular_velocity_x input double; vehicle_state_angular_velocity_y input double; vehicle_state_angular_velocity_z input double; vehicle_state_acceleration_x input double; vehicle_state_acceleration_y input double; vehicle_state_acceleration_z input double; vehicle_state_angular_acceleration_x input double; vehicle_state_angular_acceleration_y input double; vehicle_state_angular_acceleration_z input double; vehicle_state output Bus: vehicle_state
function [metadata, vehicle_state] = signals_to_bus(...
	metadata_topic, ...
	metadata_type_name, ...
	metadata_timestamp_sim_sec, ...
	metadata_timestamp_sim_nanosec, ...
	metadata_timestamp_platform_sec, ...
	metadata_timestamp_platform_nanosec, ...
	vehicle_state_state_pose_position_x, ...
	vehicle_state_state_pose_position_y, ...
	vehicle_state_state_pose_position_z, ...
	vehicle_state_state_pose_orientation_w, ...
	vehicle_state_state_pose_orientation_x, ...
	vehicle_state_state_pose_orientation_y, ...
	vehicle_state_state_pose_orientation_z, ...
	vehicle_state_velocity_x, ...
	vehicle_state_velocity_y, ...
	vehicle_state_velocity_z, ...
	vehicle_state_angular_velocity_x, ...
	vehicle_state_angular_velocity_y, ...
	vehicle_state_angular_velocity_z, ...
	vehicle_state_acceleration_x, ...
	vehicle_state_acceleration_y, ...
	vehicle_state_acceleration_z, ...
	vehicle_state_angular_acceleration_x, ...
	vehicle_state_angular_acceleration_y, ...
	vehicle_state_angular_acceleration_z )

metadata.topic = metadata_topic;
metadata.type_name = metadata_type_name;
metadata.timestamp_sim.sec = metadata_timestamp_sim_sec;
metadata.timestamp_sim.nanosec = metadata_timestamp_sim_nanosec;
metadata.timestamp_platform.sec = metadata_timestamp_platform_sec;
metadata.timestamp_platform.nanosec = metadata_timestamp_platform_nanosec;
vehicle_state.state.pose.position.x = vehicle_state_state_pose_position_x;
vehicle_state.state.pose.position.y = vehicle_state_state_pose_position_y;
vehicle_state.state.pose.position.z = vehicle_state_state_pose_position_z;
vehicle_state.state.pose.orientation.w = vehicle_state_state_pose_orientation_w;
vehicle_state.state.pose.orientation.x = vehicle_state_state_pose_orientation_x;
vehicle_state.state.pose.orientation.y = vehicle_state_state_pose_orientation_y;
vehicle_state.state.pose.orientation.z = vehicle_state_state_pose_orientation_z;
vehicle_state.velocity.x = vehicle_state_velocity_x;
vehicle_state.velocity.y = vehicle_state_velocity_y;
vehicle_state.velocity.z = vehicle_state_velocity_z;
vehicle_state.angular_velocity.x = vehicle_state_angular_velocity_x;
vehicle_state.angular_velocity.y = vehicle_state_angular_velocity_y;
vehicle_state.angular_velocity.z = vehicle_state_angular_velocity_z;
vehicle_state.acceleration.x = vehicle_state_acceleration_x;
vehicle_state.acceleration.y = vehicle_state_acceleration_y;
vehicle_state.acceleration.z = vehicle_state_acceleration_z;
vehicle_state.angular_acceleration.x = vehicle_state_angular_acceleration_x;
vehicle_state.angular_acceleration.y = vehicle_state_angular_acceleration_y;
vehicle_state.angular_acceleration.z = vehicle_state_angular_acceleration_z;

== matlab function aerosim_simulink_cosim_demo/AeroSim Output Control Signal/AeroSim JSON Encoder - Bus: simulink_out/Bus_to_Signals ==
  data: metadata input Bus: metadata; metadata_topic output string; simulink_out input Bus: simulink_out; metadata_type_name output string; metadata_timestamp_sim_sec output int32; metadata_timestamp_sim_nanosec output uint32; metadata_timestamp_platform_sec output int32; metadata_timestamp_platform_nanosec output uint32; simulink_out_control_signal_1 output double; simulink_out_main_rotor_rpm output; simulink_out_tail_rotor_rpm output
function [ ...
 metadata_topic, ...
 metadata_type_name, ...
 metadata_timestamp_sim_sec, ...
 metadata_timestamp_sim_nanosec, ...
 metadata_timestamp_platform_sec, ...
 metadata_timestamp_platform_nanosec, ...
 simulink_out_control_signal_1,...
 simulink_out_main_rotor_rpm,...
 simulink_out_tail_rotor_rpm ...
] = bus_to_signals(metadata, simulink_out)

metadata_topic = metadata.topic;
metadata_type_name = metadata.type_name;
metadata_timestamp_sim_sec = metadata.timestamp_sim.sec;
metadata_timestamp_sim_nanosec = metadata.timestamp_sim.nanosec;
metadata_timestamp_platform_sec = metadata.timestamp_platform.sec;
metadata_timestamp_platform_nanosec = metadata.timestamp_platform.nanosec;
simulink_out_control_signal_1 = simulink_out.control_signal_1;
simulink_out_main_rotor_rpm = simulink_out.main_rotor_rpm;
simulink_out_tail_rotor_rpm = simulink_out.tail_rotor_rpm;
